simulink model "model4_points"  (R2020b)
settings: Solver=VariableStepAuto  StartTime=0.0  StopTime=200  RelTol=1e-3
model workspace (MAT data in the model file):
  B = 0.169
  Kf = 0.001
  r = 0.027
undefined symbols (not defined in the file): J, ke, km, kr, ks, L, magnitude, R
settings Model: Creator=spide  LastModifiedBy=vital

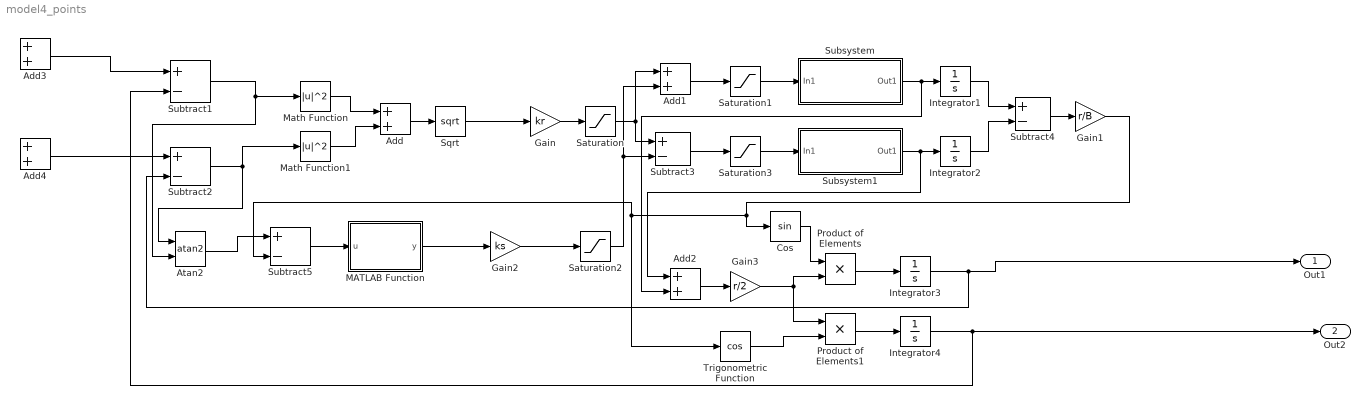
== system model4_points ==
  Add{,1..4} (5 alike) : Sum
  Atan2 : Trigonometry  Operator=atan2
  Cos : Trigonometry
  Gain : Gain  Gain=kr
  Gain1 : Gain  Gain=r/B
  Gain2 : Gain  Gain=ks
  Gain3 : Gain  Gain=r/2
  Integrator{1..4} (4 alike) : Integrator
  MATLAB Function : MATLAB Function  TreatAsAtomicUnit=on
  Math Function : Math  Operator=magnitude^2  SaturateOnIntegerOverflow=on
  Math Function1 : Math  Operator=magnitude^2  SaturateOnIntegerOverflow=on
  Product of Elements : Product  Inputs=**
  Product of Elements1 : Product  Inputs=**
  Saturation{,1..3} (4 alike) : Saturate  UpperLimit=7  LowerLimit=-7
  Sqrt : Sqrt  SaturateOnIntegerOverflow=on
  Subsystem : Subsystem
  Subsystem1 : Subsystem
  Subtract{1..5} (5 alike) : Sum  Inputs=+-
  Trigonometric Function : Trigonometry  Operator=cos
  Out1 : Outport  SignalName=Y
  Out2 : Outport  Port=2  SignalName=X
  wires:
  Math Function/1 -> Add/1
  Math Function1/1 -> Add/2
  Add/1 -> Sqrt/1
  Sqrt/1 -> Gain/1
  Gain/1 -> Saturation/1
  Saturation/1 -> Subtract3/1, Add1/1
  Add1/1 -> Saturation1/1
  Subtract3/1 -> Saturation3/1
  Saturation1/1 -> Subsystem/1(In1)
  Saturation3/1 -> Subsystem1/1(In1)
  Subsystem/1(Out1) -> Add2/2, Integrator1/1
  Integrator1/1 -> Subtract4/1
  Subsystem1/1(Out1) -> Add2/1, Integrator2/1
  Integrator2/1 -> Subtract4/2
  Subtract4/1 -> Gain1/1
  Atan2/1 -> Subtract5/1
  Gain2/1 -> Saturation2/1
  Saturation2/1 -> Subtract3/2, Add1/2
  Add2/1 -> Gain3/1
  Cos/1 -> Product of Elements/1
  Gain3/1 -> Product of Elements1/1, Product of Elements/2
  Trigonometric Function/1 -> Product of Elements1/2
  Product of Elements/1 -> Integrator3/1
  Product of Elements1/1 -> Integrator4/1
  Gain1/1 -> Subtract5/2, Trigonometric Function/1, Cos/1
  Subtract2/1 -> Math Function1/1, Atan2/1
  Subtract1/1 -> Atan2/2, Math Function/1
  Subtract5/1 -> MATLAB Function/1(u)
  MATLAB Function/1(y) -> Gain2/1
  Add3/1 -> Subtract1/1
  Add4/1 -> Subtract2/1
  Integrator4/1 -> Subtract1/2, Out2/1
  Integrator3/1 -> Out1/1, Subtract2/2

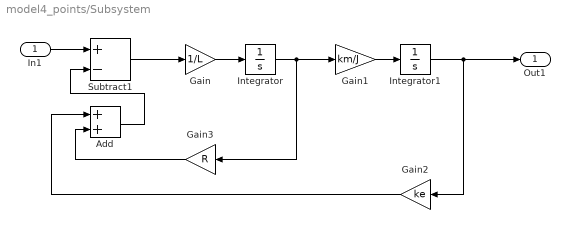
== system model4_points/Subsystem ==
  In1 : Inport
  Add : Sum
  Gain : Gain  Gain=1/L
  Gain1 : Gain  Gain=km/J
  Gain2 : Gain  Gain=ke
  Gain3 : Gain  Gain=R
  Integrator : Integrator
  Integrator1 : Integrator
  Subtract1 : Sum  Inputs=+-
  Out1 : Outport
  wires:
  In1/1 -> Subtract1/1
  Add/1 -> Subtract1/2
  Subtract1/1 -> Gain/1
  Gain/1 -> Integrator/1
  Gain3/1 -> Add/2
  Integrator/1 -> Gain3/1, Gain1/1
  Gain1/1 -> Integrator1/1
  Integrator1/1 -> Out1/1, Gain2/1
  Gain2/1 -> Add/1

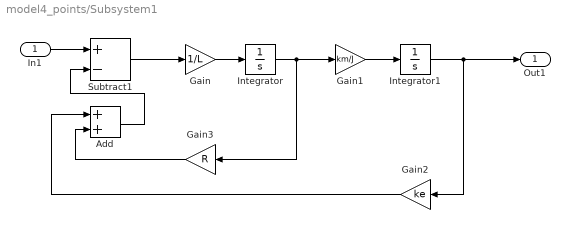
== system model4_points/Subsystem1 ==
  In1 : Inport
  Add : Sum
  Gain : Gain  Gain=1/L
  Gain1 : Gain  Gain=km/J
  Gain2 : Gain  Gain=ke
  Gain3 : Gain  Gain=R
  Integrator : Integrator
  Integrator1 : Integrator
  Subtract1 : Sum  Inputs=+-
  Out1 : Outport
  wires:
  In1/1 -> Subtract1/1
  Add/1 -> Subtract1/2
  Subtract1/1 -> Gain/1
  Gain/1 -> Integrator/1
  Gain3/1 -> Add/2
  Integrator/1 -> Gain3/1, Gain1/1
  Gain1/1 -> Integrator1/1
  Integrator1/1 -> Out1/1, Gain2/1
  Gain2/1 -> Add/1

== matlab function model4_points/MATLAB Function ==
  data: u input; y output
function y = fcn(u)
if (u > 0)
    if (abs(u) > pi)
    if (abs(u) < 2*pi)
        u = -2*pi + u;
    end
    end
elseif (u < 0)
    if (abs(u) > pi)
        if (abs(u) < 2*pi)
            u = 2*pi + u;
        end
    end
end
y = u;
